simulink model "Position_ANTTAY001"  (R2020a)
settings: Solver=ode4  StartTime=0.0  StopTime=45  FixedStep=0.2  RelTol=1e-3
undefined symbols (not defined in the file or in its folder): g, K_aug, m
settings Model: Creator=KNMALE002  LastModifiedBy=Tayla
settings DataIOCC: SaveOutput=off  SignalLogging=off  DSMLogging=off  ReturnWorkspaceOutputs=off  TimeSaveName=simulation_time
settings DebuggingCC: ArithmeticOperatorsInVariantConditions=warning
settings SFSimCC: CustomCodeUndefinedFunction=UseInterfaceOnly

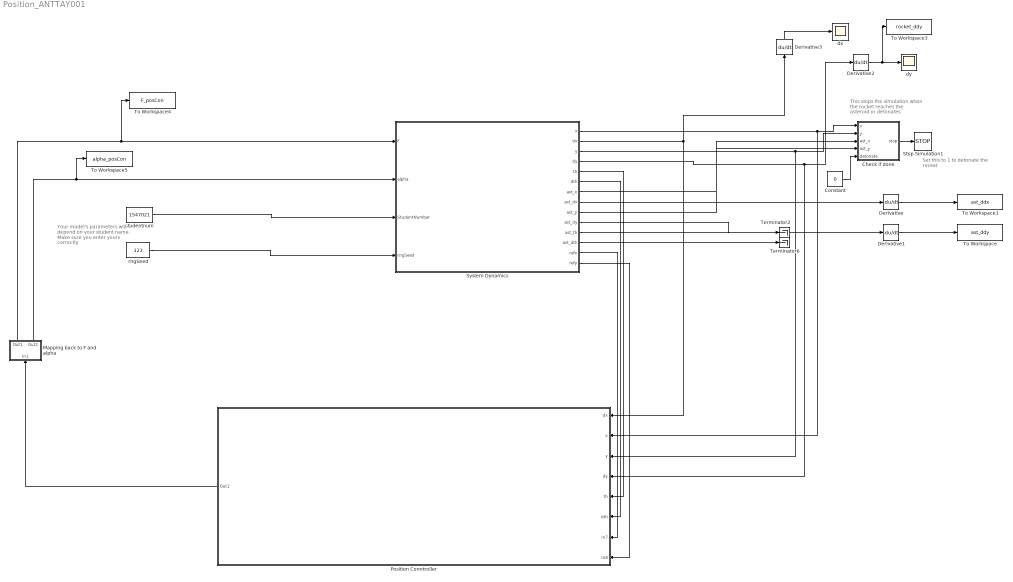
== system Position_ANTTAY001 ==
  note: Your model's parameters will depend on your student name. Make sure you enter yours correctly
  note: This stops the simulation when the rocket reaches the asteroid or detonates
  note: Set this to 1 to detonate the rocket
  Check if done : MATLAB Function  TreatAsAtomicUnit=on
  Constant : Constant  Value=0
  Derivative{,1..3} (4 alike) : Derivative
  Mapping back to F and alpha : Subsystem
  Position Conntroller : Subsystem
  Stop Simulation1 : Stop
  System Dynamics : Subsystem  TreatAsAtomicUnit=on  mask{Value=2}
      mask prompts: Value "Enter mode (1, 2 or 3)"
      mask TypeOptions Value: ScenarioVar/Value
      mask Display: image('lander.jpg');
  Terminator2 : Terminator
  Terminator6 : Terminator
  To Workspace : ToWorkspace  VariableName=ast_ddy  SampleTime=-1
  To Workspace1 : ToWorkspace  VariableName=ast_ddx  SampleTime=-1
  To Workspace3 : ToWorkspace  VariableName=rocket_ddy  SampleTime=-1
  To Workspace4 : ToWorkspace  VariableName=F_posCon  SaveFormat=Timeseries  SampleTime=-1
  To Workspace5 : ToWorkspace  VariableName=alpha_posCon  SaveFormat=Timeseries  SampleTime=-1
  dx : Scope
  dy : Scope
  rngSeed : Constant  Value=123
  studentnum : Constant  Value=1547021
  wires:
  studentnum/1 -> System Dynamics/3(StudentNumber)
  rngSeed/1 -> System Dynamics/4(rngSeed)
  System Dynamics/7(ast_x) -> Check if done/3(ast_x)
  System Dynamics/9(ast_y) -> Check if done/4(ast_y)
  Check if done/1(stop) -> Stop Simulation1/1
  Constant/1 -> Check if done/5(detonate)
  System Dynamics/8(ast_dx) -> Derivative/1
  Derivative1/1 -> To Workspace/1
  System Dynamics/10(ast_dy) -> Derivative1/1
  Derivative/1 -> To Workspace1/1
  Derivative2/1 -> To Workspace3/1, dy/1
  Derivative3/1 -> dx/1
  System Dynamics/11(ast_th) -> Terminator2/1
  System Dynamics/12(ast_dth) -> Terminator6/1
  Mapping back to F and alpha/2(Out2) -> System Dynamics/2(alpha), To Workspace5/1
  Mapping back to F and alpha/1(Out1) -> To Workspace4/1, System Dynamics/1(F)
  System Dynamics/4(dy) -> Position Conntroller/4(dy), Derivative2/1
  System Dynamics/3(y) -> Position Conntroller/3(y), Check if done/2(y)
  System Dynamics/1(x) -> Position Conntroller/2(x), Check if done/1(x)
  System Dynamics/2(dx) -> Derivative3/1, Position Conntroller/1(dx)
  System Dynamics/5(th) -> Position Conntroller/5(th)
  System Dynamics/6(dth) -> Position Conntroller/6(dth)
  System Dynamics/13(refx) -> Position Conntroller/7(In7)
  System Dynamics/14(refy) -> Position Conntroller/8(In8)
  Position Conntroller/1(Out1) -> Mapping back to F and alpha/1(In1)

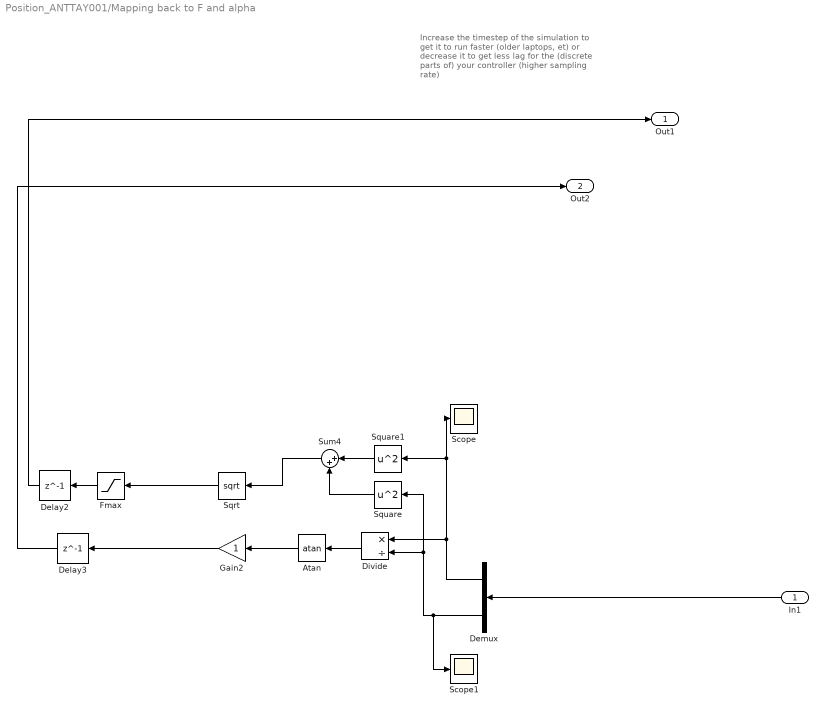
== system Position_ANTTAY001/Mapping back to F and alpha ==
  note: Increase the timestep of the simulation to get it to run faster (older laptops, et) or decrease it to get less lag for the (discrete parts of) your controller (higher sampling rate)
  In1 : Inport
  Atan : Trigonometry  Operator=atan
  Delay2 : Delay  DelayLength=1  InitialCondition=10000000000
  Delay3 : Delay  DelayLength=1
  Demux : Demux  Outputs=2
  Divide : Product  Inputs=*/
  Fmax : Saturate  UpperLimit=39250  LowerLimit=0
  Gain2 : Gain
  Scope : Scope
  Scope1 : Scope
  Sqrt : Sqrt  SaturateOnIntegerOverflow=on
  Square : Math  Operator=square  SignedPower=on  SaturateOnIntegerOverflow=on
  Square1 : Math  Operator=square  SignedPower=on  SaturateOnIntegerOverflow=on
  Sum4 : Sum  Inputs=|++
  Out1 : Outport
  Out2 : Outport  Port=2
  wires:
  Divide/1 -> Atan/1
  Demux/1 -> Divide/1, Scope/1, Square1/1
  Square1/1 -> Sum4/1
  Fmax/1 -> Delay2/1
  Demux/2 -> Scope1/1, Divide/2, Square/1
  Square/1 -> Sum4/2
  Atan/1 -> Gain2/1
  Gain2/1 -> Delay3/1
  Sum4/1 -> Sqrt/1
  Sqrt/1 -> Fmax/1
  In1/1 -> Demux/1
  Delay2/1 -> Out1/1
  Delay3/1 -> Out2/1

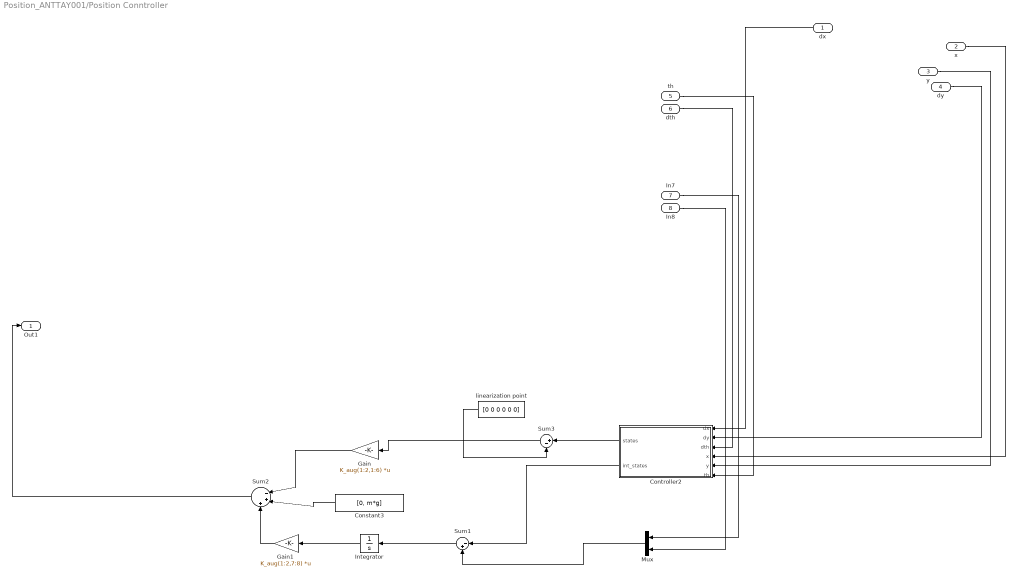
== system Position_ANTTAY001/Position Conntroller ==
  dx : Inport
  x : Inport  Port=2
  y : Inport  Port=3
  dy : Inport  Port=4
  th : Inport  Port=5
  dth : Inport  Port=6
  In7 : Inport  Port=7
  In8 : Inport  Port=8
  Constant3 : Constant  Value=[0, m*g]
  Controller2 : MATLAB Function  TreatAsAtomicUnit=on
  Gain : Gain  Gain=K_aug(1:2,1:6)  Multiplication=Matrix(K*u)
  Gain1 : Gain  Gain=K_aug(1:2,7:8)  Multiplication=Matrix(K*u)
  Integrator : Integrator
  Mux : Mux  Inputs=2
  Sum1 : Sum  Inputs=|-+
  Sum2 : Sum  Inputs=|-++
  Sum3 : Sum  Inputs=|+-
  linearization point : Constant  Value=[0 0 0 0 0 0]
  Out1 : Outport
  wires:
  Sum3/1 -> Gain/1
  Sum1/1 -> Integrator/1
  Controller2/1(states) -> Sum3/1
  Gain/1 -> Sum2/1
  Constant3/1 -> Sum2/2
  Controller2/2(int_states) -> Sum1/1
  Mux/1 -> Sum1/2
  linearization point/1 -> Sum3/2
  Gain1/1 -> Sum2/3
  Integrator/1 -> Gain1/1
  Sum2/1 -> Out1/1
  In7/1 -> Mux/1
  dy/1 -> Controller2/2(dy)
  x/1 -> Controller2/4(x)
  y/1 -> Controller2/5(y)
  th/1 -> Controller2/6(th)
  dth/1 -> Controller2/3(dth)
  In8/1 -> Mux/2
  dx/1 -> Controller2/1(dx)

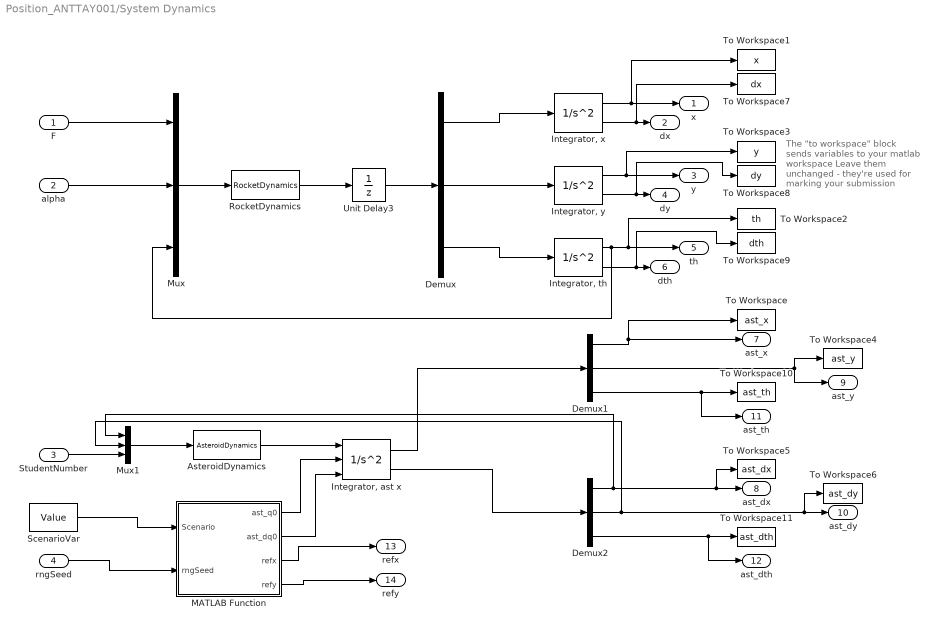
== system Position_ANTTAY001/System Dynamics ==
  note: The "to workspace" block sends variables to your matlab workspace
      |
      | Leave them unchanged - they're used for marking your submission
  F : Inport
  alpha : Inport  Port=2
  StudentNumber : Inport  Port=3
  rngSeed : Inport  Port=4
  AsteroidDynamics : MATLABFcn  MATLABFcn=AsteroidDynamics  OutputDimensions=3
  Demux : Demux  Outputs=3
  Demux1 : Demux  Outputs=3
  Demux2 : Demux  Outputs=3
  "Integrator, th" : SecondOrderIntegrator  ICX=0  ICDXDT=0
  "Integrator, x" : SecondOrderIntegrator  ICX=0
  "Integrator, y" : SecondOrderIntegrator  ICX=0
  "Integrator, ast x" : SecondOrderIntegrator  ICSourceX=external  ICX=x0  ICSourceDXDT=external
  MATLAB Function : MATLAB Function  TreatAsAtomicUnit=on
  Mux : Mux  Inputs=3
  Mux1 : Mux  Inputs=3
  RocketDynamics : MATLABFcn  MATLABFcn=RocketDynamics  Output1D=off
  ScenarioVar : Constant  Value=Value
  To Workspace : ToWorkspace  VariableName=ast_x  SampleTime=-1
  To Workspace1 : ToWorkspace  VariableName=x  SampleTime=-1
  To Workspace10 : ToWorkspace  VariableName=ast_th  SampleTime=-1
  To Workspace11 : ToWorkspace  VariableName=ast_dth  SampleTime=-1
  To Workspace2 : ToWorkspace  VariableName=th  SampleTime=-1
  To Workspace3 : ToWorkspace  VariableName=y  SampleTime=-1
  To Workspace4 : ToWorkspace  VariableName=ast_y  SampleTime=-1
  To Workspace5 : ToWorkspace  VariableName=ast_dx  SampleTime=-1
  To Workspace6 : ToWorkspace  VariableName=ast_dy  SampleTime=-1
  To Workspace7 : ToWorkspace  VariableName=dx  SampleTime=-1
  To Workspace8 : ToWorkspace  VariableName=dy  SampleTime=-1
  To Workspace9 : ToWorkspace  VariableName=dth  SampleTime=-1
  Unit Delay3 : UnitDelay  SampleTime=-1  HasFrameUpgradeWarning=on
  x : Outport  PortDimensions=1  VectorParamsAs1DForOutWhenUnconnected=off
  dx : Outport  Port=2  PortDimensions=1  VectorParamsAs1DForOutWhenUnconnected=off
  y : Outport  Port=3  PortDimensions=1  VectorParamsAs1DForOutWhenUnconnected=off
  dy : Outport  Port=4  PortDimensions=1  VectorParamsAs1DForOutWhenUnconnected=off
  th : Outport  Port=5  PortDimensions=1  VectorParamsAs1DForOutWhenUnconnected=off
  dth : Outport  Port=6  PortDimensions=1  VectorParamsAs1DForOutWhenUnconnected=off
  ast_x : Outport  Port=7  PortDimensions=1  VectorParamsAs1DForOutWhenUnconnected=off
  ast_dx : Outport  Port=8  PortDimensions=1  VectorParamsAs1DForOutWhenUnconnected=off
  ast_y : Outport  Port=9  PortDimensions=1  VectorParamsAs1DForOutWhenUnconnected=off
  ast_dy : Outport  Port=10  PortDimensions=1  VectorParamsAs1DForOutWhenUnconnected=off
  ast_th : Outport  Port=11  PortDimensions=1  VectorParamsAs1DForOutWhenUnconnected=off
  ast_dth : Outport  Port=12  PortDimensions=1  VectorParamsAs1DForOutWhenUnconnected=off
  refx : Outport  Port=13  PortDimensions=1  VectorParamsAs1DForOutWhenUnconnected=off
  refy : Outport  Port=14  PortDimensions=1  VectorParamsAs1DForOutWhenUnconnected=off
  wires:
  "Integrator, th"/1 -> th/1, To Workspace2/1, Mux/3
  Demux/1 -> "Integrator, x"/1
  Demux/2 -> "Integrator, y"/1
  Demux/3 -> "Integrator, th"/1
  "Integrator, x"/1 -> x/1, To Workspace1/1
  "Integrator, x"/2 -> To Workspace7/1, dx/1
  "Integrator, y"/2 -> To Workspace8/1, dy/1
  "Integrator, th"/2 -> To Workspace9/1, dth/1
  Mux/1 -> RocketDynamics/1
  RocketDynamics/1 -> Unit Delay3/1
  rngSeed/1 -> MATLAB Function/2(rngSeed)
  ScenarioVar/1 -> MATLAB Function/1(Scenario)
  F/1 -> Mux/1
  alpha/1 -> Mux/2
  Demux1/2 -> To Workspace4/1, ast_y/1
  Demux1/3 -> To Workspace10/1, ast_th/1
  Demux2/3 -> ast_dth/1, To Workspace11/1
  Mux1/1 -> AsteroidDynamics/1
  AsteroidDynamics/1 -> "Integrator, ast x"/1
  "Integrator, ast x"/1 -> Demux1/1
  "Integrator, ast x"/2 -> Demux2/1
  Demux1/1 -> To Workspace/1, ast_x/1
  Demux2/1 -> Mux1/1, To Workspace5/1, ast_dx/1
  Demux2/2 -> Mux1/2, To Workspace6/1, ast_dy/1
  MATLAB Function/1(ast_q0) -> "Integrator, ast x"/2
  MATLAB Function/2(ast_dq0) -> "Integrator, ast x"/3
  StudentNumber/1 -> Mux1/3
  Unit Delay3/1 -> Demux/1
  "Integrator, y"/1 -> y/1, To Workspace3/1
  MATLAB Function/3(refx) -> refx/1
  MATLAB Function/4(refy) -> refy/1

== matlab function Position_ANTTAY001/System Dynamics/MATLAB Function ==
  data: ast_q0 output; ast_dq0 output; Scenario input; rngSeed input; refx output; refy output
function [ast_q0, ast_dq0, refx, refy] = fcn(Scenario, rngSeed)
rng(rngSeed);
refx = 0;
refy = 3500;

if (Scenario == 1)
    x0 = -3000;
    y0 = 5000;
    th0 = 0;
    dx0 = 182;
    dy0 = 0;
    dth0 = 0;
    
    refx = 0;
    refy = 3500;
    
elseif (Scenario == 2)
    x0 = -2000 + rand_within_plus_minus(100);
    y0 = 4000 + rand_within_plus_minus(100);
    th0 = 0;
    dx0 = 170;
    dy0 = 0;
    dth0 = 0.1;
    
    refx = 1750;
    refy = 1600;
    theta_in = -pi/8;

elseif (Scenario == 3)
    x0 = -2500;
    y0 = 3000;
    th0 = 0;
    dx0 = 160;
    dy0 = 100;
    dth0 = deg2rad(rand_within_plus_minus(20)); % rad/sec

else
    error('You entered an invalid mode -- make sure Scenario = 1, 2 or 3')
end

ast_q0  = [ x0;  y0;  th0];
ast_dq0 = [dx0; dy0; dth0];

end

% calling rand_within_plus_minus(100) returns a number between -100 and 100
function n = rand_within_plus_minus(interval)
    n = (rand - 0.5) * 2 * interval;
end

== matlab function Position_ANTTAY001/Check if done ==
  data: x input; stop output; y input; ast_x input; ast_y input; detonate input
function stop = fcn(x, y, ast_x, ast_y, detonate)
    % given the signal to detonate
    if detonate == 1
        stop = 1;

    % rocket has hit the asteroid
    elseif norm([x; y] - [ast_x; ast_y]) < 100
        stop = 1;
    
    % rocket has hit the ground OR asteroid is close to they city
    elseif y < 0 || ast_y < 200
        stop = 1;
    
    else
        stop = 0;
    end
end

== matlab function Position_ANTTAY001/Position Conntroller/Controller2 ==
  data: dx input; dy input; dth input; states output; int_states output; x input; y input; th input
function [states, int_states] = fcn(dx, dy, dth, x, y, th)

states = [dx;dy;dth;x;y;th];
int_states = [x;y];

end
